simulink model "sim_controllo"  (R2023b)
settings: Solver=VariableStepAuto  StartTime=0.0  StopTime=10.0  RelTol=1e-3
values from neighbouring files (symbols this model uses):
  A3 = J3    [linearizzazione_controllo.m]
  B3 = double(subs(B_s,[x1,x2,u],[xeq3,ueq]))    [linearizzazione_controllo.m]
  C3 = double(subs(C_s,[x1,x2,u],[xeq3,ueq]))    [linearizzazione_controllo.m]
  ueq = 0    [linearizzazione_controllo.m]    (also in linearizzazione_non_controllo.m = 0.5)
  x0 = [3;-5]    [linearizzazione_controllo.m]    (also in linearizzazione_non_controllo.m = [0.1;6])
  xeq3 = double([xeq_s.x1(3) xeq_s.x2(3)])    [linearizzazione_controllo.m]    (also in linearizzazione_non_controllo.m)
settings Model: Creator=stefa  LastModifiedBy=stefa

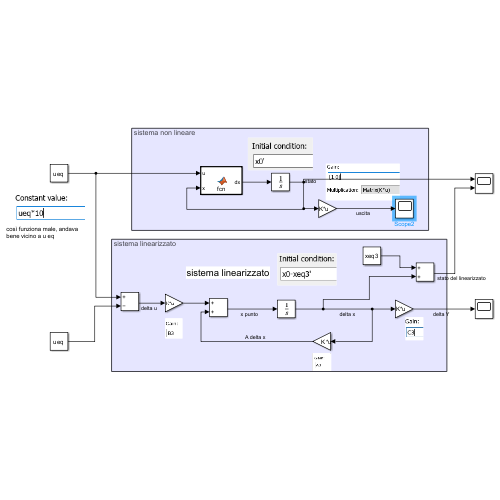
[thumbnail: Simulink's stored preview of the top-level diagram]
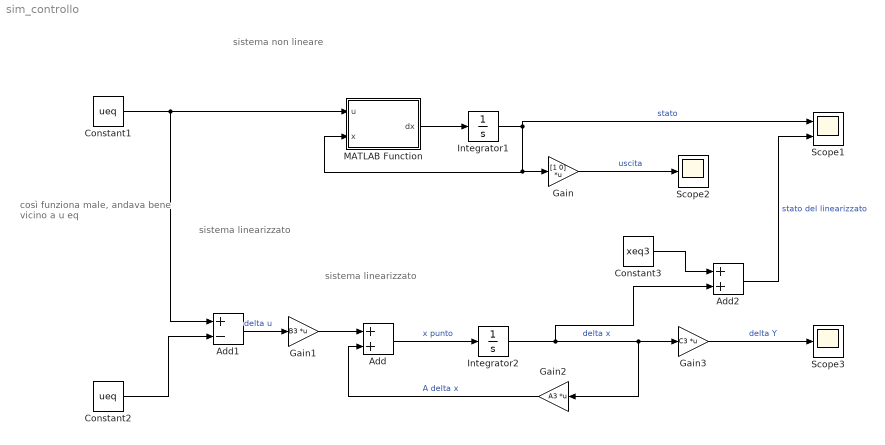
== system sim_controllo ==
  note: sistema linearizzato
  note: sistema linearizzato
  note: sistema non lineare
  note: così funziona male, andava bene vicino a u eq
  Add : Sum
  Add1 : Sum  Inputs=+-
  Add2 : Sum
  Constant1 : Constant  Value=ueq
  Constant2 : Constant  Value=ueq
  Constant3 : Constant  Value=xeq3
  Gain : Gain  Gain=[1 0]  Multiplication=Matrix(K*u)
  Gain1 : Gain  Gain=B3  Multiplication=Matrix(K*u)
  Gain2 : Gain  Gain=A3  Multiplication=Matrix(K*u)
  Gain3 : Gain  Gain=C3  Multiplication=Matrix(K*u)
  Integrator1 : Integrator  InitialCondition=x0
  Integrator2 : Integrator  InitialCondition=x0-xeq3'
  MATLAB Function : MATLAB Function  TreatAsAtomicUnit=on
  Scope1 : Scope  NumInputPorts=2
  Scope2 : Scope
  Scope3 : Scope
  wires:
  Gain3/1 -> Scope3/1  "delta Y"
  Add2/1 -> Scope1/2  "stato del linearizzato"
  Constant3/1 -> Add2/1
  Constant2/1 -> Add1/2
  MATLAB Function/1(dx) -> Integrator1/1
  Integrator1/1 -> MATLAB Function/2(x), Gain/1, Scope1/1  "stato"
  Gain1/1 -> Add/1
  Add/1 -> Integrator2/1  "x punto"
  Gain/1 -> Scope2/1  "uscita"
  Constant1/1 -> MATLAB Function/1(u), Add1/1
  Add1/1 -> Gain1/1  "delta u"
  Gain2/1 -> Add/2  "A delta x"
  Integrator2/1 -> Add2/2, Gain3/1, Gain2/1  "delta x"

== matlab function sim_controllo/MATLAB Function ==
  data: u input; dx output; x input
function dx = fcn(u,x)
x1=x(1);
x2=x(2);
dx = [-x1+6*cos(x2);(x2^2+x2)*x1-x1*u+6*cos(x1)*u];
